simulink model "grid_5bus_fdi_detection"  (R2024a)
settings: Solver=VariableStepAuto  StartTime=0.0  StopTime=4  RelTol=1e-3
libraries: spsThreePhasePISectionLineLib x7, spsThreePhaseVIMeasurementLib x5, spsLoadFlowBusLib x5, spsThreePhaseSeriesRLCLoadLib x4, spsThreePhaseFaultLib x3, spsThreePhaseSourceLib x2, spsThreePhaseProgrammableVoltageSourceLib x1, spsThreePhaseSeriesRLCBranchLib x1, spsThreePhaseBreakerLib x1, sps_lib x1
settings Model: PacingRate=0.050000  Creator=UJJWAL  LastModifiedBy=UJJWAL
settings RTWCC: GPUComputeCapability=3.5

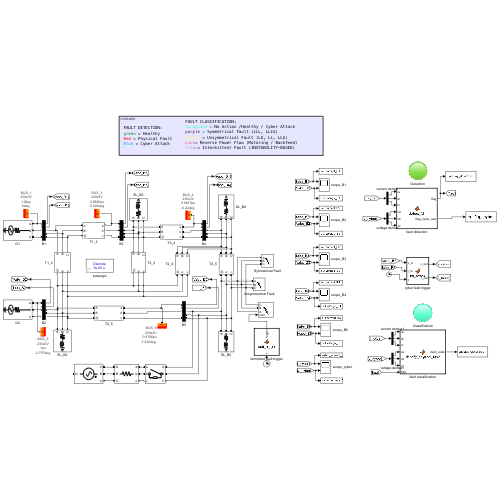
[thumbnail: Simulink's stored preview of the top-level diagram]
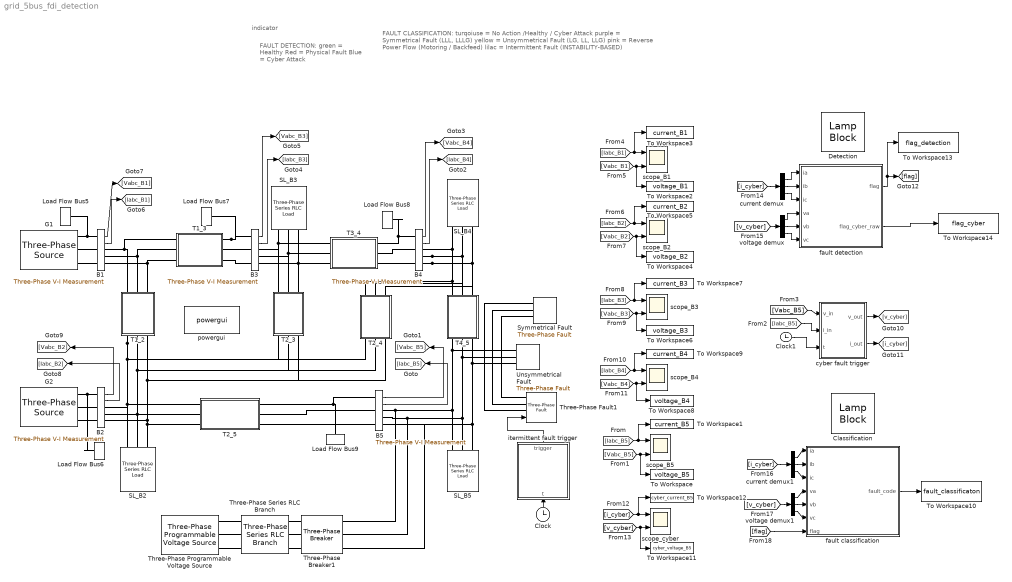
== system grid_5bus_fdi_detection ==
  note: FAULT DETECTION:
      | green = Healthy
      | Red = Physical Fault
      | Blue = Cyber Attack
  note: indicator
  note: FAULT CLASSIFICATION:
      | turqoiuse = No Action /Healthy / Cyber Attack
      | purple = Symmetrical Fault (LLL, LLLG)
      | yellow = Unsymmetrical Fault (LG, LL, LLG)
      | pink = Reverse Power Flow (Motoring / Backfeed)
      | lilac = Intermittent Fault (INSTABILITY-BASED)
  B1 : spsThreePhaseVIMeasurementLib/Three-Phase V-I Measurement  VoltageMeasurement=phase-to-ground  SetLabelV=off  LabelV=Vabc  Vpu=on  VpuLL=off  CurrentMeasurement=yes  SetLabelI=off  LabelI=Iabc  Ipu=on  Pbase=100e6  Vbase=(230000)*1.06  OutputType=Complex  PhasorSimulation=off  PSBequivalent=0
  B{2..5} (4 alike) : spsThreePhaseVIMeasurementLib/Three-Phase V-I Measurement  VoltageMeasurement=phase-to-ground  SetLabelV=off  LabelV=Vabc  Vpu=on  VpuLL=off  CurrentMeasurement=yes  SetLabelI=off  LabelI=Iabc  Ipu=on  Pbase=100e6  Vbase=230e3  OutputType=Complex  PhasorSimulation=off  PSBequivalent=0
  Classification : LampBlock  LabelPosition=Hide
  Clock : Clock
  Clock1 : Clock
  Detection : LampBlock  LabelPosition=Hide
  G1 : spsThreePhaseSourceLib/Three-Phase Source  InternalConnection=Yg  VoltagePhases=off  Voltage=(230000)*1.06  PhaseAngle=0  Voltage_phases=[25e3 25e3 25e3]/sqrt(3)  PhaseAngles_phases=[0 -120 +120]  Frequency=50  NonIdealSource=on  SpecifyImpedance=off  Resistance=1e-6  Inductance=0  ShortCircuitLevel=100e6  BaseVoltage=230e3  XRratio=7  BusType=swing  Pref=125000000  Qref=0  Prefabc=[10e3, 10e3, 10e3]  Qrefabc=[0, 0, 0]  Qmin=-300000000  Qmax=300000000
  G2 : spsThreePhaseSourceLib/Three-Phase Source  InternalConnection=Yg  VoltagePhases=off  Voltage=(230000)*1  PhaseAngle=-2.7574  Voltage_phases=[25e3 25e3 25e3]/sqrt(3)  PhaseAngles_phases=[0 -120 +120]  Frequency=50  NonIdealSource=on  SpecifyImpedance=off  Resistance=1e-6  Inductance=0  ShortCircuitLevel=100e6  BaseVoltage=230e3  XRratio=7  BusType=PV  Pref=40000000  Qref=0  Prefabc=[10e3, 10e3, 10e3]  Qrefabc=[0, 0, 0]  Qmin=-300000000  Qmax=300000000
  Load Flow Bus5 : spsLoadFlowBusLib/Load Flow Bus  LConnTagsString=a  Phases=single  Connectors=on one side  ID=BUS_1  Vbase=230e3  Vref=1.06  Vangle=0  VLF=1.06  VLFb=1  VLFc=1  angleLF=0  angleLFb=0  angleLFc=0
  Load Flow Bus6 : spsLoadFlowBusLib/Load Flow Bus  LConnTagsString=a  Phases=single  Connectors=on one side  ID=BUS_2  Vbase=230e3  Vref=1  Vangle=0  VLF=1  VLFb=1  VLFc=1  angleLF=-2.757  angleLFb=0  angleLFc=0
  Load Flow Bus7 : spsLoadFlowBusLib/Load Flow Bus  LConnTagsString=a  Phases=single  Connectors=on one side  ID=BUS_3  Vbase=230e3  Vref=1  Vangle=0  VLF=0.9865  VLFb=1  VLFc=1  angleLF=-5.822  angleLFb=0  angleLFc=0
  Load Flow Bus8 : spsLoadFlowBusLib/Load Flow Bus  LConnTagsString=a  Phases=single  Connectors=on one side  ID=BUS_4  Vbase=230e3  Vref=1  Vangle=0  VLF=0.9837  VLFb=1  VLFc=1  angleLF=-6.22  angleLFb=0  angleLFc=0
  Load Flow Bus9 : spsLoadFlowBusLib/Load Flow Bus  LConnTagsString=a  Phases=single  Connectors=on one side  ID=BUS_5  Vbase=230e3  Vref=1  Vangle=0  VLF=0.9706  VLFb=1  VLFc=1  angleLF=-7.232  angleLFb=0  angleLFc=0
  SL_B2 : spsThreePhaseSeriesRLCLoadLib/Three-Phase Series RLC Load  LConnTagsString=A|B|C  Configuration=Y (grounded)  NominalVoltage=(230000)*1  Vabc=[1e3 1e3 1e3]  Vabcp=[1e3 1e3 1e3]  NominalFrequency=50  UnbalancedPower=off  ActivePower=20000000  InductivePower=10000000  CapacitivePower=0  Pabc=[10e3 9e3 11e3]  QLabc=[100 90 110]  QCabc=[100 90 110]  Pabcp=[10e3 9e3 11e3]  QLabcp=[100 90 110]  QCabcp=[100 90 110]  Measurements=None  LoadType=constant PQ
  SL_B3 : spsThreePhaseSeriesRLCLoadLib/Three-Phase Series RLC Load  LConnTagsString=A|B|C  Configuration=Y (grounded)  NominalVoltage=(230000)*0.986531  Vabc=[1e3 1e3 1e3]  Vabcp=[1e3 1e3 1e3]  NominalFrequency=60  UnbalancedPower=off  ActivePower=45000000  InductivePower=15000000  CapacitivePower=0  Pabc=[10e3 9e3 11e3]  QLabc=[100 90 110]  QCabc=[100 90 110]  Pabcp=[10e3 9e3 11e3]  QLabcp=[100 90 110]  QCabcp=[100 90 110]  Measurements=None  LoadType=constant PQ
  SL_B4 : spsThreePhaseSeriesRLCLoadLib/Three-Phase Series RLC Load  LConnTagsString=A|B|C  Configuration=Y (grounded)  NominalVoltage=(230000)*0.983709  Vabc=[1e3 1e3 1e3]  Vabcp=[1e3 1e3 1e3]  NominalFrequency=50  UnbalancedPower=off  ActivePower=40000000  InductivePower=5000000  CapacitivePower=0  Pabc=[10e3 9e3 11e3]  QLabc=[100 90 110]  QCabc=[100 90 110]  Pabcp=[10e3 9e3 11e3]  QLabcp=[100 90 110]  QCabcp=[100 90 110]  Measurements=None  LoadType=constant PQ
  SL_B5 : spsThreePhaseSeriesRLCLoadLib/Three-Phase Series RLC Load  LConnTagsString=A|B|C  Configuration=Y (grounded)  NominalVoltage=(230000)*0.970619  Vabc=[1e3 1e3 1e3]  Vabcp=[1e3 1e3 1e3]  NominalFrequency=50  UnbalancedPower=off  ActivePower=60000000  InductivePower=10000000  CapacitivePower=0  Pabc=[10e3 9e3 11e3]  QLabc=[100 90 110]  QCabc=[100 90 110]  Pabcp=[10e3 9e3 11e3]  QLabcp=[100 90 110]  QCabcp=[100 90 110]  Measurements=None  LoadType=constant PQ
  Symmetrical Fault : spsThreePhaseFaultLib/Three-Phase Fault  InitialStates=0  FaultA=on  FaultB=on  FaultC=off  GroundFault=off  SwitchTimes=[0.25 0.35]  External=off  SwitchStatus=NaN  FaultResistance=0.001  GroundResistance=0.01  SnubberResistance=1e6  SnubberCapacitance=inf  Measurements=None
  T1_2 : Subsystem  mask{F=50, SB=100e6, V=230e3, R=0.02, X=0.06, B=0.06}
      mask prompts: F "Frequency"; SB "Base power"; V "Nominal Voltage"; R "Resistance(pu)"; X "Reactance(pu)"; B "Line Charging"
  T1_3 : Subsystem  mask{F=50, SB=100e6, V=230e3, R=0.08, X=0.24, B=0.05}
      mask prompts: F "Frequency"; SB "Base power"; V "Nominal Voltage"; R "Resistance(pu)"; X "Reactance(pu)"; B "Line Charging"
  T2_3 : Subsystem  mask{F=50, SB=100e6, V=230e3, R=0.06, X=0.18, B=0.04}
      mask prompts: F "Frequency"; SB "Base power"; V "Nominal Voltage"; R "Resistance(pu)"; X "Reactance(pu)"; B "Line Charging"
  T2_4 : Subsystem  mask{F=50, SB=100e6, V=230e3, R=0.06, X=0.18, B=0.04}
      mask prompts: F "Frequency"; SB "Base power"; V "Nominal Voltage"; R "Resistance(pu)"; X "Reactance(pu)"; B "Line Charging"
  T2_5 : Subsystem  mask{F=50, SB=100e6, V=230e3, R=0.04, X=0.12, B=0.03}
      mask prompts: F "Frequency"; SB "Base power"; V "Nominal Voltage"; R "Resistance(pu)"; X "Reactance(pu)"; B "Line Charging"
  T3_4 : Subsystem  mask{F=50, SB=100e6, V=230e3, R=0.01, X=0.03, B=0.02}
      mask prompts: F "Frequency"; SB "Base power"; V "Nominal Voltage"; R "Resistance(pu)"; X "Reactance(pu)"; B "Line Charging"
  T4_5 : Subsystem  mask{F=50, SB=100e6, V=230e3, R=0.08, X=0.24, B=0.05}
      mask prompts: F "Frequency"; SB "Base power"; V "Nominal Voltage"; R "Resistance(pu)"; X "Reactance(pu)"; B "Line Charging"
  Three-Phase Programmable Voltage Source : spsThreePhaseProgrammableVoltageSourceLib/Three-Phase Programmable Voltage Source  PositiveSequence="[230e3  0 50]"  VariationEntity=Phase  VariationType=Ramp  VariationTypeAlt=Step  VariationStep=-15  VariationRate=10  VariationMagnitude=0.3  VariationFrequency=2  VariationTiming=[0.5 0.5]  VariationPhaseA=off  Amplitudes=[1 0.8 1.2 1.0]  TimeValues=[0 0.1 0.15 0.2]  HarmonicGeneration=off  HarmonicA=[3 0.2 -25 0]  HarmonicB=[2 0.15 35 2]  Timing="[0.05  3]"  BusType=PQ  Pref=-1e6  Qref=0  Qmin=-inf  Qmax=inf
  Three-Phase Series RLC Branch : spsThreePhaseSeriesRLCBranchLib/Three-Phase Series RLC Branch  LConnTagsString=A|B|C  RConnTagsString=A|B|C  BranchType=R  Resistance=0.1  Inductance=1e-3  Capacitance=1e-6  Measurements=None
  Three-Phase Breaker1 : spsThreePhaseBreakerLib/Three-Phase Breaker  InitialState=open  SwitchA=on  SwitchB=on  SwitchC=on  SwitchTimes=[3.57 3.72]  External=off  BreakerResistance=0.01  SnubberResistance=1e6  SnubberCapacitance=inf  Measurements=None
  Three-Phase Fault1 : spsThreePhaseFaultLib/Three-Phase Fault  InitialStates=0  FaultA=on  FaultB=off  FaultC=on  GroundFault=off  SwitchTimes="[1/60  5/60]"  External=on  SwitchStatus=NaN  FaultResistance=0.001  GroundResistance=0.01  SnubberResistance=1e6  SnubberCapacitance=inf  Measurements=None
  To Workspace : ToWorkspace  VariableName=voltage_B5  SampleTime=-1
  To Workspace1 : ToWorkspace  VariableName=current_B5  SampleTime=-1
  To Workspace10 : ToWorkspace  VariableName=fault_classificaton  SampleTime=-1
  To Workspace11 : ToWorkspace  VariableName=cyber_voltage_B5  SampleTime=-1
  To Workspace12 : ToWorkspace  VariableName=cyber_current_B5  SampleTime=-1
  To Workspace13 : ToWorkspace  VariableName=flag_detection  SampleTime=-1
  To Workspace14 : ToWorkspace  VariableName=flag_cyber  SampleTime=-1
  To Workspace2 : ToWorkspace  VariableName=voltage_B1  SampleTime=-1
  To Workspace3 : ToWorkspace  VariableName=current_B1  SampleTime=-1
  To Workspace4 : ToWorkspace  VariableName=voltage_B2  SampleTime=-1
  To Workspace5 : ToWorkspace  VariableName=current_B2  SampleTime=-1
  To Workspace6 : ToWorkspace  VariableName=voltage_B3  SampleTime=-1
  To Workspace7 : ToWorkspace  VariableName=current_B3  SampleTime=-1
  To Workspace8 : ToWorkspace  VariableName=voltage_B4  SampleTime=-1
  To Workspace9 : ToWorkspace  VariableName=current_B4  SampleTime=-1
  Unsymmetrical Fault : spsThreePhaseFaultLib/Three-Phase Fault  InitialStates=0  FaultA=on  FaultB=on  FaultC=off  GroundFault=off  SwitchTimes=[2.47 2.57]  External=off  SwitchStatus=NaN  FaultResistance=0.001  GroundResistance=0.01  SnubberResistance=1e6  SnubberCapacitance=inf  Measurements=None
  current demux : Demux  Outputs=3
  current demux1 : Demux  Outputs=3
  cyber fault trigger : MATLAB Function  TreatAsAtomicUnit=on
  fault classification : MATLAB Function  TreatAsAtomicUnit=on
  fault detection : MATLAB Function  TreatAsAtomicUnit=on
  itermittent fault trigger : MATLAB Function  TreatAsAtomicUnit=on
  powergui : sps_lib/powergui  Priority=1  SimulationMode=Discrete  SampleTime=50e-6  frequency=60  Iterations=50  frequencyindice=50  Pbase=100e6  ErrMax=1e-4  UnitsV=kV  UnitsW=MW  buscounter=0  FunctionMessages=off  echomessages=off  EnableUseOfTLC=off  CurrentSourceSwitches=off  DisableSnubberDevices=off  DisableRonSwitches=off  DisableVfSwitches=off  DisplayEquations=off  AutomaticDiscreteSolvers=off  SolverType=Tustin/Backward Euler (TBE)  Interpol=off  ExternalGateDelay=off  methode=off  Ts=100  x0status=blocks  SPID=on  SwTol=0  HookPort=off  NonlinearTolerance=1e-4  nMaxIteration=100  ContinueOnMaxIteration=off  RestoreLinks=warning  ResistiveCurrentMeasurement=off  Frange=[0:2:500]  Ylog=off  Xlog=on  ShowGrid=off  save=off  variable=ZData  structure=0  ZoomFFT=off  StartTime=0.0  cycles=1  DisplayStyle=1  fundamental=60  FreqAxis=off  MaxFrequency=1000  frequencyindicesteady=1  RmsSteady=1  display=off
  scope_B{1..5} (5 alike) : Scope  NumInputPorts=2
  scope_cyber : Scope  NumInputPorts=2
  voltage demux : Demux  Outputs=3
  voltage demux1 : Demux  Outputs=3
  wires:
  [Vabc_B3] -> To Workspace6/1, scope_B3/2
  voltage demux1/3 -> fault classification/6(vc)
  B2/1 -> [Vabc_B2]
  B5/2 -> [Iabc_B5]
  B4/1 -> [Vabc_B4]
  B5/1 -> [Vabc_B5]
  B2/2 -> [Iabc_B2]
  B3/1 -> [Vabc_B3]
  [Iabc_B5] -> cyber fault trigger/2(i_in)
  cyber fault trigger/1(v_out) -> [v_cyber]
  voltage demux1/2 -> fault classification/5(vb)
  [Vabc_B1] -> To Workspace2/1, scope_B1/2
  voltage demux/2 -> fault detection/5(vb)
  B1/1 -> [Vabc_B1]
  [Iabc_B5] -> scope_B5/1, To Workspace1/1
  [flag] -> fault classification/7(flag)
  voltage demux/3 -> fault detection/6(vc)
  [Vabc_B5] -> cyber fault trigger/1(v_in)
  [i_cyber] -> current demux/1
  [v_cyber] -> voltage demux1/1
  [Iabc_B1] -> scope_B1/1, To Workspace3/1
  current demux/1 -> fault detection/1(ia)
  fault detection/1(flag) -> To Workspace13/1, [flag]
  [Iabc_B3] -> scope_B3/1, To Workspace7/1
  voltage demux/1 -> fault detection/4(va)
  Clock1/1 -> cyber fault trigger/3(t)
  current demux1/1 -> fault classification/1(ia)
  B4/2 -> [Iabc_B4]
  [i_cyber] -> scope_cyber/1, To Workspace12/1
  B1/2 -> [Iabc_B1]
  [Iabc_B4] -> scope_B4/1, To Workspace9/1
  [Vabc_B2] -> To Workspace4/1, scope_B2/2
  [Vabc_B4] -> To Workspace8/1, scope_B4/2
  current demux1/2 -> fault classification/2(ib)
  current demux1/3 -> fault classification/3(ic)
  [Iabc_B2] -> scope_B2/1, To Workspace5/1
  current demux/3 -> fault detection/3(ic)
  [Vabc_B5] -> To Workspace/1, scope_B5/2
  current demux/2 -> fault detection/2(ib)
  [i_cyber] -> current demux1/1
  [v_cyber] -> To Workspace11/1, scope_cyber/2
  B3/2 -> [Iabc_B3]
  voltage demux1/1 -> fault classification/4(va)
  [v_cyber] -> voltage demux/1
  cyber fault trigger/2(i_out) -> [i_cyber]
  itermittent fault trigger/1(trigger) -> Three-Phase Fault1/1
  Clock/1 -> itermittent fault trigger/1(t)
  fault classification/1(fault_code) -> To Workspace10/1
  fault detection/2(flag_cyber_raw) -> To Workspace14/1
  connections:
  B4/RConn2 -- T2_4/LConn2 -- T4_5/LConn2 -- SL_B4/LConn2
  T2_4/LConn1 -- T4_5/LConn1 -- SL_B4/LConn1 -- B4/RConn1
  SL_B3/LConn1 -- T2_3/LConn1 -- B3/RConn1 -- T3_4/LConn1
  SL_B3/LConn2 -- T2_3/LConn2 -- B3/RConn2 -- T3_4/LConn2
  T1_3/RConn1 -- Load Flow Bus7/LConn1 -- B3/LConn1
  Three-Phase Breaker1/LConn2 -- B5/RConn2 -- Three-Phase Fault1/LConn2 -- Unsymmetrical Fault/LConn2 -- Symmetrical Fault/LConn2 -- T4_5/RConn2 -- SL_B5/LConn2
  T1_2/LConn1 -- T1_3/LConn1 -- B1/RConn1
  SL_B5/LConn3 -- B5/RConn3 -- Three-Phase Breaker1/LConn3 -- Three-Phase Fault1/LConn3 -- Unsymmetrical Fault/LConn3 -- Symmetrical Fault/LConn3 -- T4_5/RConn3
  Load Flow Bus8/LConn1 -- B4/LConn1 -- T3_4/RConn1
  T1_2/LConn3 -- T1_3/LConn3 -- B1/RConn3
  SL_B2/LConn2 -- T2_5/LConn2 -- B2/RConn2 -- T2_3/RConn2 -- T2_4/RConn2 -- T1_2/RConn2
  T1_2/LConn2 -- T1_3/LConn2 -- B1/RConn2
  T3_4/LConn3 -- T2_3/LConn3 -- SL_B3/LConn3 -- B3/RConn3
  SL_B2/LConn3 -- T2_5/LConn3 -- B2/RConn3 -- T2_4/RConn3 -- T2_3/RConn3 -- T1_2/RConn3
  T1_2/RConn1 -- T2_5/LConn1 -- B2/RConn1 -- SL_B2/LConn1 -- T2_4/RConn1 -- T2_3/RConn1
  B4/RConn3 -- SL_B4/LConn3 -- T2_4/LConn3 -- T4_5/LConn3
  Load Flow Bus9/LConn1 -- B5/LConn1 -- T2_5/RConn1
  B5/RConn1 -- Three-Phase Breaker1/LConn1 -- Unsymmetrical Fault/LConn1 -- Three-Phase Fault1/LConn1 -- Symmetrical Fault/LConn1 -- T4_5/RConn1 -- SL_B5/LConn1
  G2/RConn1 -- Load Flow Bus6/LConn1 -- B2/LConn1
  Load Flow Bus5/LConn1 -- B1/LConn1 -- G1/RConn1
  Three-Phase Programmable Voltage Source/RConn1 -- Three-Phase Series RLC Branch/LConn3
  B5/LConn3 -- T2_5/RConn3
  B4/LConn3 -- T3_4/RConn3
  B3/LConn3 -- T1_3/RConn3
  Three-Phase Series RLC Branch/RConn3 -- Three-Phase Breaker1/RConn3
  Three-Phase Series RLC Branch/RConn1 -- Three-Phase Breaker1/RConn1
  B2/LConn2 -- G2/RConn2
  B3/LConn2 -- T1_3/RConn2
  B4/LConn2 -- T3_4/RConn2
  Three-Phase Programmable Voltage Source/RConn3 -- Three-Phase Series RLC Branch/LConn1
  B5/LConn2 -- T2_5/RConn2
  B1/LConn2 -- G1/RConn2
  B1/LConn3 -- G1/RConn3
  Three-Phase Series RLC Branch/RConn2 -- Three-Phase Breaker1/RConn2
  Three-Phase Programmable Voltage Source/RConn2 -- Three-Phase Series RLC Branch/LConn2
  B2/LConn3 -- G2/RConn3

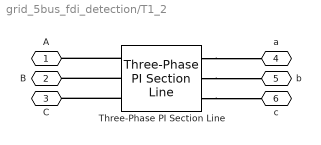
== system grid_5bus_fdi_detection/T1_2 ==
  Three-Phase PI Section Line : spsThreePhasePISectionLineLib/Three-Phase PI Section Line  LConnTagsString=a|b|c  RConnTagsString=A|B|C  Length=floor((3e5)*(sqrt(X*B))/(2*pi*F))  Frequency=F  Resistances=[ (R*(V^2)/SB)/floor((3e5)*(sqrt(X*B))/(2*pi*F)) 3*(R*(V^2)/SB)/floor((3e5)*(sqrt(X*B))/(2*pi*F))]  Inductances=[ (X*(V^2)/SB)/(2*pi*F*floor((3e5)*(sqrt(X*B))/(2*pi*F))) 3*(X*(V^2)/SB)/(2*pi*F*floor((3e5)*(sqrt(X*B))/(2*pi*F)))]  Capacitances=[(B*SB)/((floor((3e5)*(sqrt(X*B))/(2*pi*F)))*2*pi*F*V^2) (3*B*SB)/((floor((3e5)*(sqrt(X*B))/(2*pi*F)))*2*pi*F*V^2)]
  A : PMIOPort  Side=Left
  B : PMIOPort  Port=2  Side=Left
  C : PMIOPort  Port=3  Side=Left
  a : PMIOPort  Port=4  Side=Right
  b : PMIOPort  Port=5  Side=Right
  c : PMIOPort  Port=6  Side=Right
  connections:
  Three-Phase PI Section Line/RConn1 -- a/RConn1
  Three-Phase PI Section Line/LConn3 -- C/RConn1
  Three-Phase PI Section Line/LConn1 -- A/RConn1
  Three-Phase PI Section Line/RConn3 -- c/RConn1
  Three-Phase PI Section Line/RConn2 -- b/RConn1
  Three-Phase PI Section Line/LConn2 -- B/RConn1

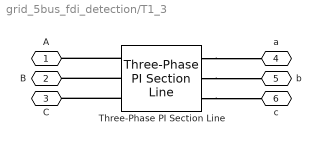
== system grid_5bus_fdi_detection/T1_3 ==
  Three-Phase PI Section Line : spsThreePhasePISectionLineLib/Three-Phase PI Section Line  LConnTagsString=a|b|c  RConnTagsString=A|B|C  Length=floor((3e5)*(sqrt(X*B))/(2*pi*F))  Frequency=F  Resistances=[ (R*(V^2)/SB)/floor((3e5)*(sqrt(X*B))/(2*pi*F)) 3*(R*(V^2)/SB)/floor((3e5)*(sqrt(X*B))/(2*pi*F))]  Inductances=[ (X*(V^2)/SB)/(2*pi*F*floor((3e5)*(sqrt(X*B))/(2*pi*F))) 3*(X*(V^2)/SB)/(2*pi*F*floor((3e5)*(sqrt(X*B))/(2*pi*F)))]  Capacitances=[(B*SB)/((floor((3e5)*(sqrt(X*B))/(2*pi*F)))*2*pi*F*V^2) (3*B*SB)/((floor((3e5)*(sqrt(X*B))/(2*pi*F)))*2*pi*F*V^2)]
  A : PMIOPort  Side=Left
  B : PMIOPort  Port=2  Side=Left
  C : PMIOPort  Port=3  Side=Left
  a : PMIOPort  Port=4  Side=Right
  b : PMIOPort  Port=5  Side=Right
  c : PMIOPort  Port=6  Side=Right
  connections:
  Three-Phase PI Section Line/LConn2 -- B/RConn1
  Three-Phase PI Section Line/RConn2 -- b/RConn1
  Three-Phase PI Section Line/RConn3 -- c/RConn1
  Three-Phase PI Section Line/LConn1 -- A/RConn1
  Three-Phase PI Section Line/LConn3 -- C/RConn1
  Three-Phase PI Section Line/RConn1 -- a/RConn1

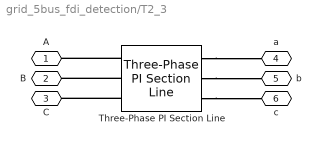
== system grid_5bus_fdi_detection/T2_3 ==
  Three-Phase PI Section Line : spsThreePhasePISectionLineLib/Three-Phase PI Section Line  LConnTagsString=a|b|c  RConnTagsString=A|B|C  Length=floor((3e5)*(sqrt(X*B))/(2*pi*F))  Frequency=F  Resistances=[ (R*(V^2)/SB)/floor((3e5)*(sqrt(X*B))/(2*pi*F)) 3*(R*(V^2)/SB)/floor((3e5)*(sqrt(X*B))/(2*pi*F))]  Inductances=[ (X*(V^2)/SB)/(2*pi*F*floor((3e5)*(sqrt(X*B))/(2*pi*F))) 3*(X*(V^2)/SB)/(2*pi*F*floor((3e5)*(sqrt(X*B))/(2*pi*F)))]  Capacitances=[(B*SB)/((floor((3e5)*(sqrt(X*B))/(2*pi*F)))*2*pi*F*V^2) (3*B*SB)/((floor((3e5)*(sqrt(X*B))/(2*pi*F)))*2*pi*F*V^2)]
  A : PMIOPort  Side=Left
  B : PMIOPort  Port=2  Side=Left
  C : PMIOPort  Port=3  Side=Left
  a : PMIOPort  Port=4  Side=Right
  b : PMIOPort  Port=5  Side=Right
  c : PMIOPort  Port=6  Side=Right
  connections:
  Three-Phase PI Section Line/LConn2 -- B/RConn1
  Three-Phase PI Section Line/RConn2 -- b/RConn1
  Three-Phase PI Section Line/RConn3 -- c/RConn1
  Three-Phase PI Section Line/LConn1 -- A/RConn1
  Three-Phase PI Section Line/LConn3 -- C/RConn1
  Three-Phase PI Section Line/RConn1 -- a/RConn1

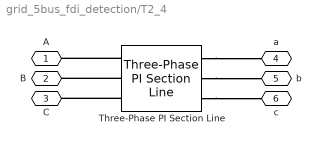
== system grid_5bus_fdi_detection/T2_4 ==
  Three-Phase PI Section Line : spsThreePhasePISectionLineLib/Three-Phase PI Section Line  LConnTagsString=a|b|c  RConnTagsString=A|B|C  Length=floor((3e5)*(sqrt(X*B))/(2*pi*F))  Frequency=F  Resistances=[ (R*(V^2)/SB)/floor((3e5)*(sqrt(X*B))/(2*pi*F)) 3*(R*(V^2)/SB)/floor((3e5)*(sqrt(X*B))/(2*pi*F))]  Inductances=[ (X*(V^2)/SB)/(2*pi*F*floor((3e5)*(sqrt(X*B))/(2*pi*F))) 3*(X*(V^2)/SB)/(2*pi*F*floor((3e5)*(sqrt(X*B))/(2*pi*F)))]  Capacitances=[(B*SB)/((floor((3e5)*(sqrt(X*B))/(2*pi*F)))*2*pi*F*V^2) (3*B*SB)/((floor((3e5)*(sqrt(X*B))/(2*pi*F)))*2*pi*F*V^2)]
  A : PMIOPort  Side=Left
  B : PMIOPort  Port=2  Side=Left
  C : PMIOPort  Port=3  Side=Left
  a : PMIOPort  Port=4  Side=Right
  b : PMIOPort  Port=5  Side=Right
  c : PMIOPort  Port=6  Side=Right
  connections:
  Three-Phase PI Section Line/RConn1 -- a/RConn1
  Three-Phase PI Section Line/LConn3 -- C/RConn1
  Three-Phase PI Section Line/LConn1 -- A/RConn1
  Three-Phase PI Section Line/RConn3 -- c/RConn1
  Three-Phase PI Section Line/RConn2 -- b/RConn1
  Three-Phase PI Section Line/LConn2 -- B/RConn1

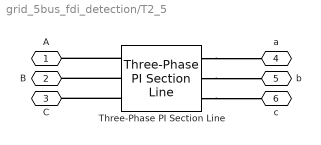
== system grid_5bus_fdi_detection/T2_5 ==
  Three-Phase PI Section Line : spsThreePhasePISectionLineLib/Three-Phase PI Section Line  LConnTagsString=a|b|c  RConnTagsString=A|B|C  Length=floor((3e5)*(sqrt(X*B))/(2*pi*F))  Frequency=F  Resistances=[ (R*(V^2)/SB)/floor((3e5)*(sqrt(X*B))/(2*pi*F)) 3*(R*(V^2)/SB)/floor((3e5)*(sqrt(X*B))/(2*pi*F))]  Inductances=[ (X*(V^2)/SB)/(2*pi*F*floor((3e5)*(sqrt(X*B))/(2*pi*F))) 3*(X*(V^2)/SB)/(2*pi*F*floor((3e5)*(sqrt(X*B))/(2*pi*F)))]  Capacitances=[(B*SB)/((floor((3e5)*(sqrt(X*B))/(2*pi*F)))*2*pi*F*V^2) (3*B*SB)/((floor((3e5)*(sqrt(X*B))/(2*pi*F)))*2*pi*F*V^2)]
  A : PMIOPort  Side=Left
  B : PMIOPort  Port=2  Side=Left
  C : PMIOPort  Port=3  Side=Left
  a : PMIOPort  Port=4  Side=Right
  b : PMIOPort  Port=5  Side=Right
  c : PMIOPort  Port=6  Side=Right
  connections:
  Three-Phase PI Section Line/LConn2 -- B/RConn1
  Three-Phase PI Section Line/RConn2 -- b/RConn1
  Three-Phase PI Section Line/RConn3 -- c/RConn1
  Three-Phase PI Section Line/LConn1 -- A/RConn1
  Three-Phase PI Section Line/LConn3 -- C/RConn1
  Three-Phase PI Section Line/RConn1 -- a/RConn1

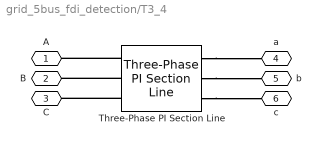
== system grid_5bus_fdi_detection/T3_4 ==
  Three-Phase PI Section Line : spsThreePhasePISectionLineLib/Three-Phase PI Section Line  LConnTagsString=a|b|c  RConnTagsString=A|B|C  Length=floor((3e5)*(sqrt(X*B))/(2*pi*F))  Frequency=F  Resistances=[ (R*(V^2)/SB)/floor((3e5)*(sqrt(X*B))/(2*pi*F)) 3*(R*(V^2)/SB)/floor((3e5)*(sqrt(X*B))/(2*pi*F))]  Inductances=[ (X*(V^2)/SB)/(2*pi*F*floor((3e5)*(sqrt(X*B))/(2*pi*F))) 3*(X*(V^2)/SB)/(2*pi*F*floor((3e5)*(sqrt(X*B))/(2*pi*F)))]  Capacitances=[(B*SB)/((floor((3e5)*(sqrt(X*B))/(2*pi*F)))*2*pi*F*V^2) (3*B*SB)/((floor((3e5)*(sqrt(X*B))/(2*pi*F)))*2*pi*F*V^2)]
  A : PMIOPort  Side=Left
  B : PMIOPort  Port=2  Side=Left
  C : PMIOPort  Port=3  Side=Left
  a : PMIOPort  Port=4  Side=Right
  b : PMIOPort  Port=5  Side=Right
  c : PMIOPort  Port=6  Side=Right
  connections:
  Three-Phase PI Section Line/RConn1 -- a/RConn1
  Three-Phase PI Section Line/LConn3 -- C/RConn1
  Three-Phase PI Section Line/LConn1 -- A/RConn1
  Three-Phase PI Section Line/RConn3 -- c/RConn1
  Three-Phase PI Section Line/RConn2 -- b/RConn1
  Three-Phase PI Section Line/LConn2 -- B/RConn1

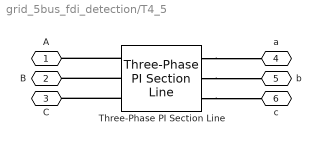
== system grid_5bus_fdi_detection/T4_5 ==
  Three-Phase PI Section Line : spsThreePhasePISectionLineLib/Three-Phase PI Section Line  LConnTagsString=a|b|c  RConnTagsString=A|B|C  Length=floor((3e5)*(sqrt(X*B))/(2*pi*F))  Frequency=F  Resistances=[ (R*(V^2)/SB)/floor((3e5)*(sqrt(X*B))/(2*pi*F)) 3*(R*(V^2)/SB)/floor((3e5)*(sqrt(X*B))/(2*pi*F))]  Inductances=[ (X*(V^2)/SB)/(2*pi*F*floor((3e5)*(sqrt(X*B))/(2*pi*F))) 3*(X*(V^2)/SB)/(2*pi*F*floor((3e5)*(sqrt(X*B))/(2*pi*F)))]  Capacitances=[(B*SB)/((floor((3e5)*(sqrt(X*B))/(2*pi*F)))*2*pi*F*V^2) (3*B*SB)/((floor((3e5)*(sqrt(X*B))/(2*pi*F)))*2*pi*F*V^2)]
  A : PMIOPort  Side=Left
  B : PMIOPort  Port=2  Side=Left
  C : PMIOPort  Port=3  Side=Left
  a : PMIOPort  Port=4  Side=Right
  b : PMIOPort  Port=5  Side=Right
  c : PMIOPort  Port=6  Side=Right
  connections:
  Three-Phase PI Section Line/LConn2 -- B/RConn1
  Three-Phase PI Section Line/RConn2 -- b/RConn1
  Three-Phase PI Section Line/RConn3 -- c/RConn1
  Three-Phase PI Section Line/LConn1 -- A/RConn1
  Three-Phase PI Section Line/LConn3 -- C/RConn1
  Three-Phase PI Section Line/RConn1 -- a/RConn1

== matlab function grid_5bus_fdi_detection/fault detection ==
  data: ia input; ib input; ic input; va input; flag output; vb input; vc input; flag_cyber_raw output
function [flag, flag_cyber_raw] = detect_fdi(ia, ib, ic, va, vb, vc)
% detect_fdi  Fault and FDI (False Data Injection) detection for 3-phase systems.
%
%   Outputs:
%     flag           - 0: normal | 1: cyber attack | 2: physical fault (Prioritised)
%     flag_cyber_raw - 0: no cyber | 1: cyber attack (Independent, not overridden by physical)
%     Z_out          - instantaneous impedance estimate
%     Irms_out       - per-phase RMS current (proxy)
%     Vrms_out       - per-phase RMS voltage (proxy)
eps_val = 1e-6;

% -------- PERSISTENT STATES --------
persistent prev_flag cyber_count fault_count fault_latch dir_integral ...
           prev_va prev_vb prev_vc frozen_count ...
           prev_ia prev_ib prev_ic noise_buf_idx noise_var_buf ...
           is_rpf_active cyber_holdoff 

if isempty(prev_flag)
    prev_flag     = 0;
    cyber_count   = 0;
    fault_count   = 0;
    fault_latch   = 0;
    dir_integral  = 0;
    prev_va       = 0; prev_vb = 0; prev_vc = 0;
    frozen_count  = 0;
    prev_ia       = 0; prev_ib = 0; prev_ic = 0;
    noise_buf_idx = 1;
    noise_var_buf = zeros(1, 20);
    is_rpf_active = false;
    cyber_holdoff = 0;
end

% -------- RMS & POWER CALCULATIONS --------
Vrms  = sqrt((va^2 + vb^2 + vc^2) / 3);
Irms  = sqrt((ia^2 + ib^2 + ic^2) / 3);
Z     = Vrms / (Irms + eps_val);
P     = va*ia + vb*ib + vc*ic;
P_mag = abs(P);

% ==========================================
% 1. THRESHOLDS (normalised per-unit values)
% ==========================================
Z_mean_base = 1.7702;
I_mean_base = 0.3882;
V_mean_base = 0.6872;

Z_upper    = 1.25 * Z_mean_base;
Z_lower    = 0.75 * Z_mean_base;
I_fault_th = 1.30 * I_mean_base;   
I_hif_th   = 0.70 * I_mean_base;   

% ==========================================
% 2. PHYSICS / CYBER VOLTAGE BOUNDARY
% ==========================================
is_phys_voltage  = (Vrms <  0.985 * V_mean_base);
is_cyber_voltage = (Vrms >= 0.985 * V_mean_base);

% ==========================================
% 3. PHYSICAL FAULT DETECTION (Magnitudes)
% ==========================================
short_fault = (Z < Z_lower)  && (Irms > I_fault_th) && is_phys_voltage;
hif_fault   = (Z > Z_upper)  && (Irms < I_hif_th)   && is_phys_voltage;

% ==========================================
% 4. CYBER TRAP CONDITIONS (Modes 4 & 5)
% ==========================================
fake_hif   = (Z > Z_upper) && (Irms < I_hif_th)    && is_cyber_voltage;
fake_short = (Z < Z_lower) && (Irms > I_fault_th)  && is_cyber_voltage;
fake_sag   = (Vrms < 0.95 * V_mean_base) && (Irms > 0.5 * I_mean_base) && is_cyber_voltage;
fake_swell = (Vrms > 1.05 * V_mean_base) && (Irms > I_hif_th)          && is_cyber_voltage;

% Replay attack: voltage samples frozen
delta_v = abs(va - prev_va) + abs(vb - prev_vb) + abs(vc - prev_vc);
if delta_v < 1e-3
    frozen_count = frozen_count + 1;
else
    frozen_count = 0;
end
replay_attack = (frozen_count > 5);

% Noise injection attack
dI = abs(ia - prev_ia) + abs(ib - prev_ib) + abs(ic - prev_ic);
noise_var_buf(noise_buf_idx) = dI^2;
noise_buf_idx = mod(noise_buf_idx, 20) + 1;
noise_attack  = (mean(noise_var_buf) > (20 * (0.02 * I_mean_base)^2));

% Breaker-open detection
is_breaker_open = (Irms < 0.30 * I_mean_base);

% Consolidated cyber condition
cyber_cond = fake_hif   || fake_short || fake_sag   || fake_swell || ...
             replay_attack || noise_attack || (P_mag > 3.0);

% ==========================================
% 5. PHYSICAL FAULT TIMER & INTEGRAL RPF
% ==========================================
% --- Track A: Magnitude Fault Timer ---
if (short_fault || hif_fault)
    fault_count = fault_count + 1;
else
    fault_count = 0;
end
phys_fault_detected = (fault_count >= 3);

% --- Track B: Reverse Power Flow Integrator ---
Ts = 50e-6; 
dir_integral = dir_integral + (sign(P) * Ts);

% Guarded, Gentler Fast Decay
is_normal_mags = (Vrms >= 0.985 * V_mean_base) && (Irms < I_fault_th);
if is_normal_mags && (fault_latch == 0) && (dir_integral < 0)
    dir_integral = dir_integral + (1 * Ts); 
end
if dir_integral > 0 
    dir_integral = 0; 
end   

% RPF Hysteresis Latch
if dir_integral <= -0.015
    is_rpf_active = true;  
elseif dir_integral == 0
    is_rpf_active = false; 
end

% --- Simultaneous Decision ---
fault_detected = phys_fault_detected || is_rpf_active;

% ==========================================
% 6. CYBER EVENT COUNTER & BLANKING
% ==========================================
% Manage the internal blanking timer
if fault_detected
    cyber_holdoff = 200; % 10ms blanking for physical recovery ringing
elseif cyber_holdoff > 0
    cyber_holdoff = cyber_holdoff - 1;
end

% Block cyber accumulation during dead-bus or recovery holdoff
if is_breaker_open || (cyber_holdoff > 0)
    cyber_count = 0;
    noise_var_buf(:) = 0; % Flushes the noise buffer
    frozen_count = 0;
elseif cyber_cond
    if fake_hif || fake_short || fake_sag || fake_swell
        cyber_count = cyber_count + 5;
    else
        cyber_count = cyber_count + 2;
    end
else
    cyber_count = max(0, cyber_count - 5);
end

cyber_detected = (cyber_count >= 10);

% ==========================================
% 7. FINAL DECISION (Prioritised Output)
% ==========================================
if fault_detected
    flag        = 2;
    fault_latch = 250;  
elseif fault_latch > 0
    fault_latch = fault_latch - 1;
    flag        = 2;
elseif cyber_detected && ~is_breaker_open
    flag = 1;
else
    flag = 0;
end

% ==========================================
% 8. INDEPENDENT CYBER FLAG (Unfiltered Output)
% ==========================================
% This flag goes high if a cyber attack is detected, regardless of 
% whether a physical fault is currently active and overriding the main 'flag'.
if cyber_detected && ~is_breaker_open
    flag_cyber_raw = 1;
else
    flag_cyber_raw = 0;
end

% -------- UPDATE PERSISTENT STATE --------
prev_ia   = ia;  prev_ib = ib;  prev_ic = ic;
prev_va   = va;  prev_vb = vb;  prev_vc = vc;
prev_flag = flag;   

end

== matlab function grid_5bus_fdi_detection/itermittent fault trigger ==
  data: t input; trigger output
function trigger = fault_trigger(t)
    trigger = 0;
    
    % Intermittent arcing fault: 6 Spikes (20ms ON, 20ms OFF)
    % Updated specifically for the 4-second simulation timeline
    intervals = [
        2.49 2.51;  % Spike 1
        2.53 2.55;  % Spike 2
        2.57 2.59;  % Spike 3
        2.61 2.63;  % Spike 4
        2.65 2.67;  % Spike 5
        2.69 2.71   % Spike 6
    ];
    
    for i = 1:size(intervals,1)
        if t >= intervals(i,1) && t <= intervals(i,2)
            trigger = 1;
            return;
        end
    end
end

== matlab function grid_5bus_fdi_detection/cyber fault trigger ==
  settings: updateMethod=DISCRETE
  data: v_in input; i_in input; v_out output; t input; i_out output
function [v_out, i_out] = fdi_attack(v_in, i_in, t)
%#codegen
persistent stored_v stored_i attack_active

if isempty(stored_v)
    stored_v = v_in;
    stored_i = i_in;
    attack_active = false;
end

% -------- DEFAULT OUTPUT --------
v_out = v_in;
i_out = i_in;

% -------- TIME-BASED ATTACK WINDOWS (4-SECOND TIMELINE) --------

if (t >= 0.750) && (t <= 0.950)
    % EVENT 2: PURE CYBER ATTACK (Scaling Attack)
    scale_factor = 1.5;
    v_out = scale_factor * v_in;
    i_out = scale_factor * i_in;
    
elseif (t >= 1.300) && (t <= 1.520)
    % EVENT 3: UNSYM FAULT + CYBER (Replay Attack)
    if ~attack_active
        % Grabs the signal exactly at t = 1.300s and replays it
        stored_v = v_in;
        stored_i = i_in;
        attack_active = true;
    end
    v_out = stored_v;
    i_out = stored_i;
    
elseif (t >= 1.870) && (t <= 2.120)
    % EVENT 4: RPF + CYBER (Current Manipulation)
    v_out = v_in;
    
    % Split behavior at the exact midpoint of this specific window (1.995s)
    if t < 1.995
        i_out = 0.5 * i_in;   % Fake HIF
    else
        i_out = 1.8 * i_in;   % Overload
    end
    
elseif (t >= 2.470) && (t <= 2.810)
    % EVENT 5: INTERMITTENT + CYBER (Voltage Manipulation)
    i_out = i_in;
    
    % Split behavior at the exact midpoint of this specific window (2.640s)
    if t < 2.640
        v_out = 0.5 * v_in;   % Fake Voltage Sag
    else
        v_out = 1.8 * v_in;   % Fake Voltage Swell
    end
    
elseif (t >= 3.160) && (t <= 3.360)
    % EVENT 6: EXTRA PURE CYBER (Bias Attack)
    % Shifted to fit before the 4.000s simulation end
    bias = 0.2;
    v_out = v_in + bias;
    i_out = i_in + bias;
    
else
    % -------- OUTSIDE ALL ATTACK WINDOWS --------
    % Passing normal values and resetting the replay attack trigger
    v_out = v_in;
    i_out = i_in;
    attack_active = false; 
end

end

== matlab function grid_5bus_fdi_detection/fault classification ==
  data: ia input; ib input; ic input; va input; vb input; vc input; fault_code output; flag input
function fault_code = classify_physical_fault(ia, ib, ic, va, vb, vc, flag)
    eps_val = 1e-6;

    persistent prev_flag fluct_count fluct_timer intermittent_latch ...
               dir_integral is_rpf_active rpf_event_latch ...
               ia_buf ib_buf ic_buf rms_buf_idx

    if isempty(prev_flag);          prev_flag          = 0;     end
    if isempty(fluct_count);        fluct_count        = 0;     end
    if isempty(fluct_timer);        fluct_timer        = 0;     end
    if isempty(intermittent_latch); intermittent_latch = 0;     end
    if isempty(dir_integral);       dir_integral       = 0;     end
    if isempty(is_rpf_active);      is_rpf_active      = false; end
    if isempty(rpf_event_latch);    rpf_event_latch    = false; end

    cycle_len = 400;
    if isempty(ia_buf);      ia_buf      = zeros(1, cycle_len); end
    if isempty(ib_buf);      ib_buf      = zeros(1, cycle_len); end
    if isempty(ic_buf);      ic_buf      = zeros(1, cycle_len); end
    if isempty(rms_buf_idx); rms_buf_idx = 1;                   end

    fault_code = 0;

    % ── 1. Rolling one-cycle RMS ─────────────────────────────────────────
    ia_buf(rms_buf_idx) = ia^2;
    ib_buf(rms_buf_idx) = ib^2;
    ic_buf(rms_buf_idx) = ic^2;
    rms_buf_idx = mod(rms_buf_idx, cycle_len) + 1;

    Ia_rms = sqrt(mean(ia_buf));
    Ib_rms = sqrt(mean(ib_buf));
    Ic_rms = sqrt(mean(ic_buf));

    % ── 2. Intermittent fault tracker ───────────────────────────────────
    fluct_window = 4000;
    if fluct_timer > 0
        fluct_timer = fluct_timer - 1;
    end
    
    if (flag == 2) && (prev_flag ~= 2)
        fluct_count = fluct_count + 1;
        fluct_timer = fluct_window;
    end
    prev_flag = flag;

    if fluct_count >= 3
        intermittent_latch = 1;
    end

    % Guard against spurious reset when timer expires while flag==2
    if (fluct_timer == 0) && (fluct_count > 0) && (flag ~= 2)
        fluct_count        = 0;
        intermittent_latch = 0;
    end

    % ── 3. Reverse power tracker ─────────────────────────────────────────
    Ts = 50e-6;
    P  = va*ia + vb*ib + vc*ic;
    dir_integral = dir_integral + (sign(P) * Ts);

    if (flag ~= 2) && (dir_integral < 0)
        dir_integral = dir_integral + (1 * Ts);
    end
    
    if dir_integral > 0
        dir_integral = 0;
    end

    if dir_integral <= -0.015
        is_rpf_active   = true;
        rpf_event_latch = true;
    elseif dir_integral == 0
        is_rpf_active = false;
    end

    if (flag == 2) && (dir_integral <= -0.004)
        rpf_event_latch = true;
    end

    % ── 4. Absolute priority — intermittent fault ────────────────────────
    if intermittent_latch == 1
        fault_code = 4;
        return;
    end

    % ── 5. Gatekeeper — physical fault only ─────────────────────────────
    if flag ~= 2
        rpf_event_latch = false;
        return;
    end

    % ── 6. Priority fault overrides ──────────────────────────────────────
    if rpf_event_latch
        fault_code = 3;
        return;
    end

    % ── 7. Symmetrical vs unsymmetrical ──────────────────────────────────
    I_avg_rms = (Ia_rms + Ib_rms + Ic_rms) / 3;
    unbalance = max([abs(Ia_rms - I_avg_rms), ...
                     abs(Ib_rms - I_avg_rms), ...
                     abs(Ic_rms - I_avg_rms)]) / (I_avg_rms + eps_val);

    if unbalance > 0.15
        fault_code = 2;
    else
        fault_code = 1;
    end
end
